simulink model "Subsystem"  (R2020a)
settings: Solver=VariableStepAuto  StartTime=0.0  StopTime=120  RelTol=1e-3
undefined symbols (not defined in the file or in its folder): b, D, I, m, P
settings Model: DataDictionary=ModelData.sldd  Creator=tnradm  LastModifiedBy=tnradm
settings DataIOCC: SaveOutput=off  SaveTime=off

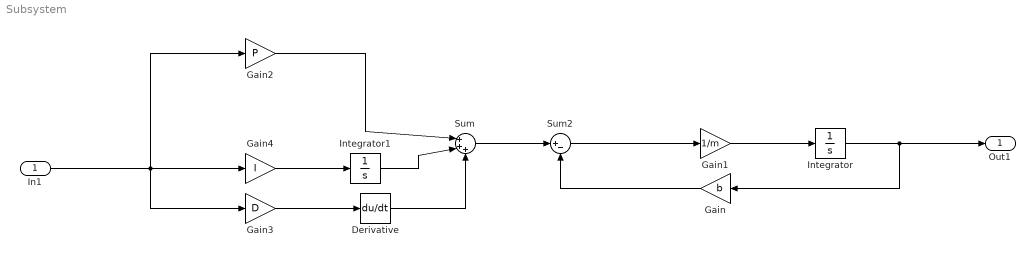
== system Subsystem ==
  In1 : Inport  OutDataTypeStr=double  PortDimensions=1  SampleTime=0
  Derivative : Derivative
  Gain : Gain  Gain=b
  Gain1 : Gain  Gain=1/m
  Gain2 : Gain  Gain=P
  Gain3 : Gain  Gain=D
  Gain4 : Gain  Gain=I
  Integrator : Integrator
  Integrator1 : Integrator
  Sum : Sum  Inputs=|+++
  Sum2 : Sum  Inputs=|+-
  Out1 : Outport  OutDataTypeStr=double  PortDimensions=1  SampleTime=0
  wires:
  Integrator1/1 -> Sum/2
  Gain4/1 -> Integrator1/1
  Integrator/1 -> Gain/1, Out1/1
  Sum/1 -> Sum2/1
  Gain2/1 -> Sum/1
  In1/1 -> Gain4/1, Gain3/1, Gain2/1
  Derivative/1 -> Sum/3
  Gain3/1 -> Derivative/1
  Gain1/1 -> Integrator/1
  Sum2/1 -> Gain1/1
  Gain/1 -> Sum2/2
